simulink model "SimDraft3"  (R2024b)
settings: Solver=VariableStepAuto  StartTime=0.0  StopTime=2  RelTol=1e-3
model workspace (MAT data in the model file):
  CanaryAmplitude = 1
  CanaryCarrierFrequency = 20000
  CanaryDataRate = 100
  DataAmplitude = 1
  SampleRate = 44100
  SoundSpeed = 300
undefined symbols (not defined in the file or in its folder): magnitude
libraries: commseqgen3 x4, dspfdesign x3, audiosources x2, dspstat3 x2, simulink x2, dspsigops x2, commchan3 x1
settings Model: PacingRate=0.007100  Creator=calum  LastModifiedBy=calum
settings OptimizationCC: StateBitsets=on  DataBitsets=on  AccelVerboseBuild=on
settings ModelReferenceCC: UpdateModelReferenceTargets=IfOutOfDate  EnableParallelModelReferenceBuilds=on  ParallelModelReferenceMATLABWorkerInit=Copy Base Workspace
settings SFSimCC: SimHardwareAcceleration=native

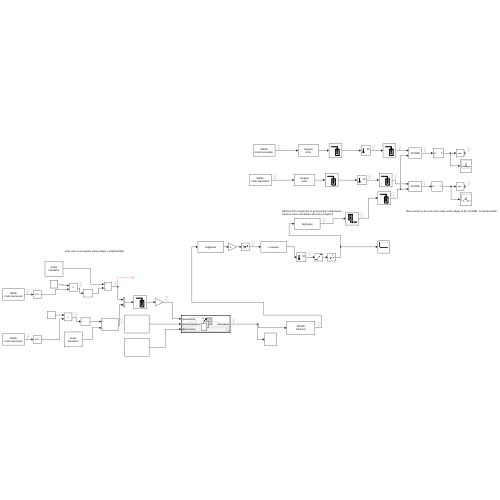
[thumbnail: Simulink's stored preview of the top-level diagram]
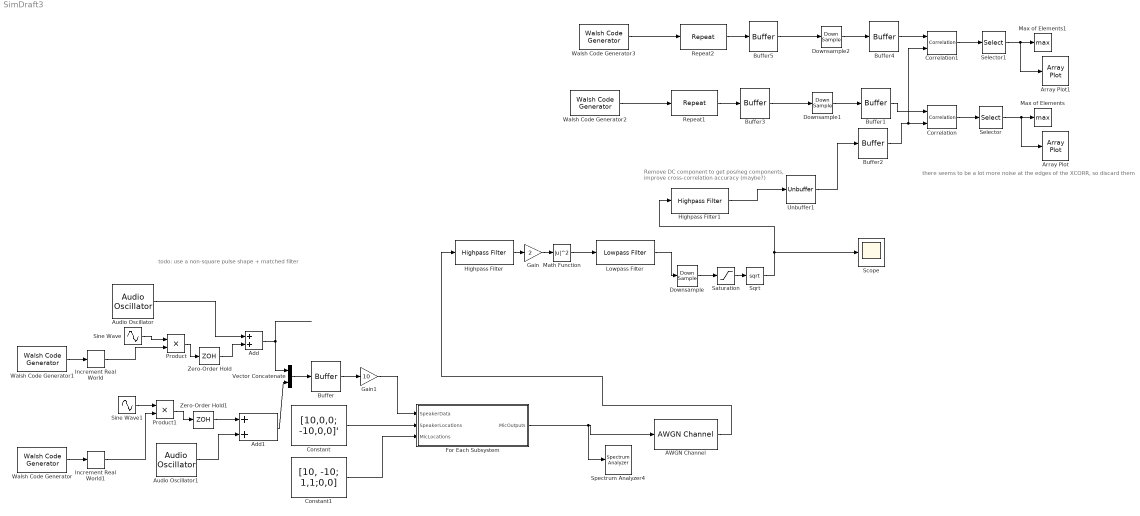
== system SimDraft3 ==
  note: there seems to be a lot more noise at the edges of the XCORR, so discard them
  note: Remove DC component to get pos/neg components,
      | improve cross-correlation accuracy (maybe?)
  note: todo: use a non-square pulse shape + matched filter
  AWGN Channel : commchan3/AWGN Channel  LegacyMode=off  NoiseMethod="Signal to noise ratio  (SNR)"  noiseMode="Signal to noise ratio  (SNR)"  EbNo=10  EsNo=10  SNR=200  BitsPerSymbol=1  SignalPower=1  SamplesPerSymbol=1  SymbolPeriod=1  VarianceSource=Parameter  Variance=1  RandomStream=Global stream  Seed=67  SimulateUsing=Code generation
  Add : Sum
  Add1 : Sum
  Array Plot : ArrayPlot  WindowPosition=[106.000000,368.000000,1454.000000,673.000000,]  ScopeFrameLocation=window  YLimits=[-4297.499458035714 3899.8950419642856]  ShowLegend=on
  Array Plot1 : ArrayPlot  WindowPosition=[106.000000,368.000000,1454.000000,673.000000,]  ScopeFrameLocation=window  YLimits=[-4018.8112 4055.0609]  ShowLegend=on
  Audio Oscillator : audiosources/Audio Oscillator  FrequencyPort=off  Frequency=200  AmplitudePort=off  Amplitude=DataAmplitude  DCOffsetPort=off  DCOffset=0  PhaseOffset=0  WidthPort=off  Width=1  DutyCyclePort=off  DutyCycle=0.5  SampsPerFrame=1  Fs=SampleRate  OutputDataType=double  SimulateUsing=Code generation
      settings: SignalType=sine
  Audio Oscillator1 : audiosources/Audio Oscillator  FrequencyPort=off  Frequency=400  AmplitudePort=off  Amplitude=DataAmplitude  DCOffsetPort=off  DCOffset=0  PhaseOffset=0  WidthPort=off  Width=1  DutyCyclePort=off  DutyCycle=0.5  SampsPerFrame=1  Fs=SampleRate  OutputDataType=double  SimulateUsing=Code generation
      settings: SignalType=sine
  Buffer : Buffer  OutputFrames=off
  Buffer1 : Buffer  N=ceil(SampleRate/32/CanaryDataRate*16)  V=220  OutputFrames=off
  Buffer2 : Buffer  N=ceil(SampleRate/32/CanaryDataRate*32)+10  V=ceil(SampleRate/32/CanaryDataRate*32)+9  OutputFrames=off
  Buffer3 : Buffer  N=32  OutputFrames=off
  Buffer4 : Buffer  N=ceil(SampleRate/32/CanaryDataRate*16)  OutputFrames=off
  Buffer5 : Buffer  N=32  OutputFrames=off
  Constant : Constant  Value="[10,0,0;  -10,0,0]'"
  Constant1 : Constant  Value=[10, -10; 1,1;0,0]
  Correlation : dspstat3/Correlation  domain=Time  roundingMode=Floor  overflowMode=off  outputDataTypeStr=Inherit: Same as accumulator  outputMin=[]  outputMax=[]  outputLastDataTypeStr=Inherit: Same as accumulator
  Correlation1 : dspstat3/Correlation  domain=Time  roundingMode=Floor  overflowMode=off  outputDataTypeStr=Inherit: Same as accumulator  outputMin=[]  outputMax=[]  outputLastDataTypeStr=Inherit: Same as accumulator
  Downsample : DownSample  N=32
  Downsample1 : DownSample  N=32
  Downsample2 : DownSample  N=32
  For Each Subsystem : Subsystem  TreatAsAtomicUnit=on
  Gain : Gain  Gain=2
  Gain1 : Gain  Gain=10
  Highpass Filter : dspfdesign/Highpass Filter  FilterType=FIR  DesignForMinimumOrder=on  FilterOrder=50  StopbandFrequency=CanaryCarrierFrequency-20*CanaryDataRate  PassbandFrequency=CanaryCarrierFrequency-3*CanaryDataRate  StopbandAttenuation=80  PassbandRipple=2  SampleRateMode=Specify on dialog  SampleRate=SampleRate  SimulateUsing=Code generation  roundingMode=Floor  coeffsDataTypeStr=fixdt(1,16)
  Highpass Filter1 : dspfdesign/Highpass Filter  FilterType=FIR  DesignForMinimumOrder=on  FilterOrder=50  StopbandFrequency=1  PassbandFrequency=CanaryDataRate  StopbandAttenuation=80  PassbandRipple=0.1  SampleRateMode=Specify on dialog  SampleRate=SampleRate  SimulateUsing=Code generation  roundingMode=Floor  coeffsDataTypeStr=fixdt(1,16)
  Increment Real World : simulink/Additional Math & Discrete/Additional Math: Increment - Decrement/Increment Real World
  Increment Real World1 : simulink/Additional Math & Discrete/Additional Math: Increment - Decrement/Increment Real World
  Lowpass Filter : dspfdesign/Lowpass Filter  FilterType=FIR  DesignForMinimumOrder=on  FilterOrder=50  PassbandFrequency=CanaryDataRate*2  StopbandFrequency=CanaryDataRate*20  PassbandRipple=0.1  StopbandAttenuation=80  SampleRateMode=Specify on dialog  SampleRate=44100  SimulateUsing=Code generation  roundingMode=Floor  coeffsDataTypeStr=fixdt(1,16)
  Math Function : Math  Operator=magnitude^2
  Max of Elements : MinMax  Function=max  CollapseMode=Specified dimension
  Max of Elements1 : MinMax  Function=max  CollapseMode=Specified dimension
  Product : Product
  Product1 : Product
  Repeat1 : dspsigops/Repeat  FactorSource=Dialog parameter  N=SampleRate/CanaryDataRate  Nmax=16  InputProcessing=Columns as channels (frame based)  RateOptions=Allow multirate processing  ic=0  mode=Unused parameter value
      settings: LibrarySourceBlock=commsequence2/Repeat
  Repeat2 : dspsigops/Repeat  FactorSource=Dialog parameter  N=SampleRate/CanaryDataRate  Nmax=16  InputProcessing=Columns as channels (frame based)  RateOptions=Allow multirate processing  ic=0  mode=Unused parameter value
      settings: LibrarySourceBlock=commsequence2/Repeat
  Saturation : Saturate  UpperLimit=inf  LowerLimit=0
  Scope : Scope
  Selector : Selector  NumberOfDimensions=2  InputPortWidth=3  IndexOptions=Index vector (dialog),Select all  Indices=[225 : 225+221],1  OutputSizes=1,1
  Selector1 : Selector  NumberOfDimensions=2  InputPortWidth=3  IndexOptions=Index vector (dialog),Select all  Indices=[225 : 225+221],1  OutputSizes=1,1
  Sine Wave : Sin  Amplitude=CanaryAmplitude  Frequency=2*pi*CanaryCarrierFrequency  SampleTime=0
  Sine Wave1 : Sin  Amplitude=CanaryAmplitude  Frequency=2*pi*CanaryCarrierFrequency  SampleTime=0
  Spectrum Analyzer4 : SpectrumAnalyzer  WindowPosition=[1.000000,38.000000,1920.000000,1003.000000,]  ScopeFrameLocation=window  SampleRateSource=Property  SampleRate=44.1e3  PlotAsTwoSidedSpectrum=off  FrequencyScale=Log  FrequencySpan=Start and stop frequencies  StartFrequency=20  StopFrequency=20e3  YLimits=[-35.36873114,56.89093674]
  Sqrt : Sqrt
  Unbuffer1 : Unbuffer
  Vector Concatenate : Concatenate  Mode=Multidimensional array  ConcatenateDimension=2
  Walsh Code Generator : commseqgen3/Walsh Code Generator  Length=16  Index=9  SampleTime=1/CanaryDataRate  SamplesPerFrame=1  OutputDataType=double  SimulateUsing=Code generation
  Walsh Code Generator1 : commseqgen3/Walsh Code Generator  Length=16  Index=3  SampleTime=1/CanaryDataRate  SamplesPerFrame=1  OutputDataType=double  SimulateUsing=Code generation
  Walsh Code Generator2 : commseqgen3/Walsh Code Generator  Length=16  Index=3  SampleTime=1/CanaryDataRate  SamplesPerFrame=1  OutputDataType=double  SimulateUsing=Code generation
  Walsh Code Generator3 : commseqgen3/Walsh Code Generator  Length=16  Index=9  SampleTime=1/CanaryDataRate  SamplesPerFrame=1  OutputDataType=double  SimulateUsing=Code generation
  Zero-Order Hold : ZeroOrderHold  SampleTime=1/SampleRate
  Zero-Order Hold1 : ZeroOrderHold  SampleTime=1/SampleRate
  wires:
  Vector Concatenate/1 -> Buffer/1
  Sine Wave/1 -> Product/1
  Sine Wave1/1 -> Product1/1
  Walsh Code Generator/1 -> Increment Real World1/1
  Product/1 -> Zero-Order Hold/1
  Audio Oscillator/1 -> Add/1
  Add/1 -> Vector Concatenate/1
  Add1/1 -> Vector Concatenate/2
  Product1/1 -> Zero-Order Hold1/1
  Audio Oscillator1/1 -> Add1/2
  Zero-Order Hold/1 -> Add/2
  Zero-Order Hold1/1 -> Add1/1
  Buffer/1 -> Gain1/1
  Walsh Code Generator1/1 -> Increment Real World/1
  AWGN Channel/1 -> Highpass Filter/1
  Lowpass Filter/1 -> Downsample/1
  Gain/1 -> Math Function/1
  Sqrt/1 -> Highpass Filter1/1, Scope/1
  Highpass Filter/1 -> Gain/1
  Gain1/1 -> For Each Subsystem/1(SpeakerData)
  For Each Subsystem/1(MicOutputs) -> Spectrum Analyzer4/1, AWGN Channel/1
  Constant/1 -> For Each Subsystem/2(SpeakerLocations)
  Constant1/1 -> For Each Subsystem/3(MicLocations)
  Increment Real World/1 -> Product/2
  Increment Real World1/1 -> Product1/2
  Downsample/1 -> Saturation/1
  Math Function/1 -> Lowpass Filter/1
  Buffer1/1 -> Correlation/1
  Buffer2/1 -> Correlation1/2, Correlation/2
  Downsample1/1 -> Buffer1/1
  Correlation/1 -> Selector/1
  Repeat1/1 -> Buffer3/1
  Buffer3/1 -> Downsample1/1
  Unbuffer1/1 -> Buffer2/1
  Saturation/1 -> Sqrt/1
  Highpass Filter1/1 -> Unbuffer1/1
  Walsh Code Generator2/1 -> Repeat1/1
  Walsh Code Generator3/1 -> Repeat2/1
  Repeat2/1 -> Buffer5/1
  Buffer5/1 -> Downsample2/1
  Downsample2/1 -> Buffer4/1
  Buffer4/1 -> Correlation1/1
  Correlation1/1 -> Selector1/1
  Selector/1 -> Max of Elements/1, Array Plot/1
  Selector1/1 -> Max of Elements1/1, Array Plot1/1

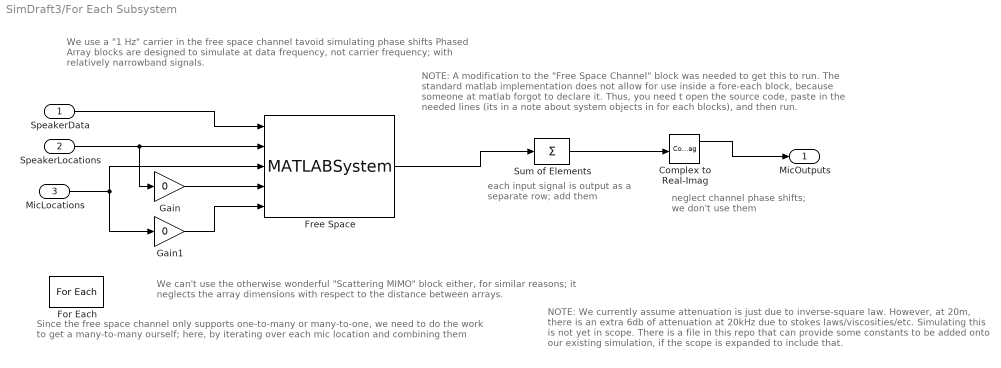
== system SimDraft3/For Each Subsystem ==
  note: NOTE: We currently assume attenuation is just due to inverse-square law.
      | However, at 20m, there is an extra 6db of attenuation at 20kHz due to stokes laws/viscosities/etc.  Simulating this is not yet in scope.  There is a file in this repo that can provide some constants to be added onto our existing simulation, if the scope is expanded to include that.
  note: neglect channel phase
      | shifts; we don't use them
  note: each input signal is output as
      | a separate row; add them
  note: NOTE: A modification to the "Free Space Channel" block was needed to get
      | this to run.  The standard matlab implementation does not allow for use inside a fore-each block, because someone at matlab forgot to declare it.  Thus, you need t open the source code, paste in the needed lines (its in a note about system objects in for each blocks), and then run.
  note: Since the free space channel only supports one-to-many or many-to-one, we need to do the work to get a many-to-many ourself; here, by iterating over each mic location and combining them
  note: We can't use the otherwise wonderful "Scattering MIMO" block either, for similar reasons;
      | it neglects the array dimensions with respect to the distance between arrays.
  note: We use a "1 Hz" carrier in the free space channel tavoid simulating phase shifts
      | Phased Array blocks are designed to simulate at data frequency, not carrier frequency;
      | with relatively narrowband signals.
  SpeakerData : Inport
  SpeakerLocations : Inport  Port=2
  MicLocations : Inport  Port=3  Partition=on  PartitionDimension=2  PartitionWidth=1  PartitionOffset=0
  Complex to Real-Imag : ComplexToRealImag
  For Each : ForEach  DisableCoverage=on
  Free Space : MATLABSystem  System=FreeSpaceCalum  PropagationSpeed=SoundSpeed  OperatingFrequency=0.000001  TwoWayPropagation=off  SampleRateFromInputCheckbox=on  SampleRate=1e6  MaximumDistanceSource=Property  MaximumDistance=10e3  MaximumNumInputSamplesSource=Auto  MaximumNumInputSamples=100  SimulateUsing=Code generation
      settings: LibrarySourceBlock=phasedenvlib/Free Space
  Gain : Gain  Gain=0
  Gain1 : Gain  Gain=0
  Sum of Elements : Sum  Inputs=+  CollapseMode=Specified dimension  CollapseDim=2
  MicOutputs : Outport  ConcatenationDimension=2
  wires:
  SpeakerData/1 -> Free Space/1
  SpeakerLocations/1 -> Free Space/2, Gain/1
  Free Space/1 -> Sum of Elements/1
  Sum of Elements/1 -> Complex to Real-Imag/1
  Gain/1 -> Free Space/4
  Gain1/1 -> Free Space/5
  MicLocations/1 -> Gain1/1, Free Space/3
  Complex to Real-Imag/1 -> MicOutputs/1
